simulink model "W2problem4"  (R2021a)
settings: Solver=VariableStepAuto  StartTime=0.0  StopTime=10.0  RelTol=1e-3
undefined symbols (not defined in the file): b, J, Ke, Kt, L, R
settings Model: Creator=Nida  LastModifiedBy=Nida

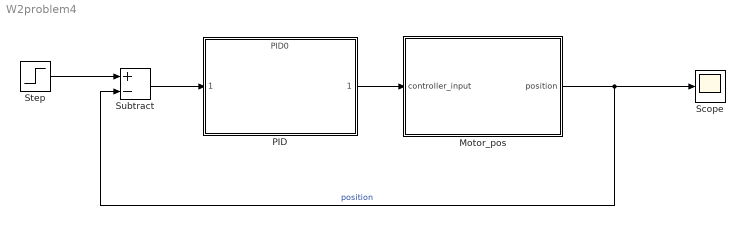
== system W2problem4 ==
  Motor_pos : Subsystem
  PID : ModelReference  ModelNameDialog=PID0  SimulationMode=Normal  ModelReferenceVersion=2.1
  Scope : Scope
  Step : Step  SampleTime=0
  Subtract : Sum  Inputs=+-
  wires:
  Motor_pos/1(position) -> Subtract/2, Scope/1  "position"
  Step/1 -> Subtract/1
  Subtract/1 -> PID/1
  PID/1 -> Motor_pos/1(controller_input)

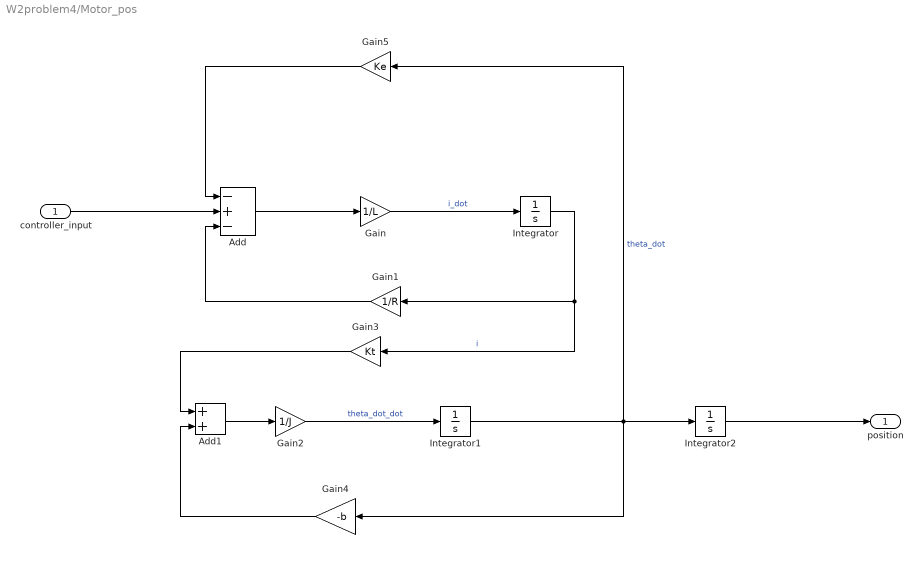
== system W2problem4/Motor_pos ==
  controller_input : Inport
  Add : Sum  Inputs=-+-
  Add1 : Sum
  Gain : Gain  Gain=1/L
  Gain1 : Gain  Gain=1/R
  Gain2 : Gain  Gain=1/J
  Gain3 : Gain  Gain=Kt
  Gain4 : Gain  Gain=-b
  Gain5 : Gain  Gain=Ke
  Integrator : Integrator
  Integrator1 : Integrator
  Integrator2 : Integrator
  position : Outport
  wires:
  Add1/1 -> Gain2/1
  controller_input/1 -> Add/2
  Gain/1 -> Integrator/1  "i_dot"
  Integrator/1 -> Gain1/1, Gain3/1  "i"
  Gain3/1 -> Add1/1
  Gain1/1 -> Add/3
  Integrator1/1 -> Integrator2/1, Gain5/1, Gain4/1  "theta_dot"
  Add/1 -> Gain/1
  Integrator2/1 -> position/1
  Gain4/1 -> Add1/2
  Gain2/1 -> Integrator1/1  "theta_dot_dot"
  Gain5/1 -> Add/1
